simulink model "Single_phase_unipolar_mf39"  (R2023b)
settings: Solver=ode45  StartTime=0.0  StopTime=0.1  RelTol=1e-3
libraries: spsDiodeLib x4, spsIdealSwitchLib x4, spsCurrentMeasurementLib x1, spsDCVoltageSourceLib x1, spsSeriesRLCBranchLib x1, spsTriangleGeneratorLib x1, spsVoltageMeasurementLib x1, spspowerguiLib x1
settings Model: Creator=LX  LastModifiedBy=Ngsanchong
settings DataIOCC: ReturnWorkspaceOutputs=off

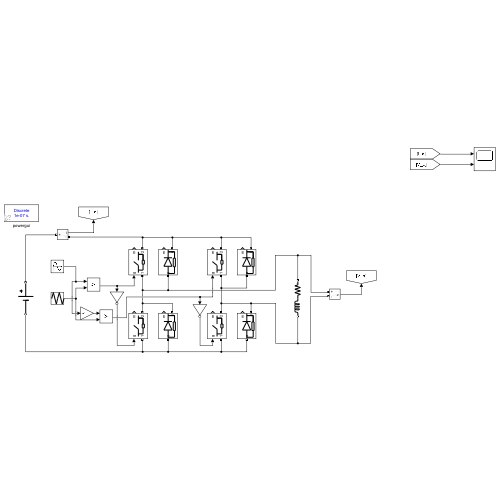
[thumbnail: Simulink's stored preview of the top-level diagram]
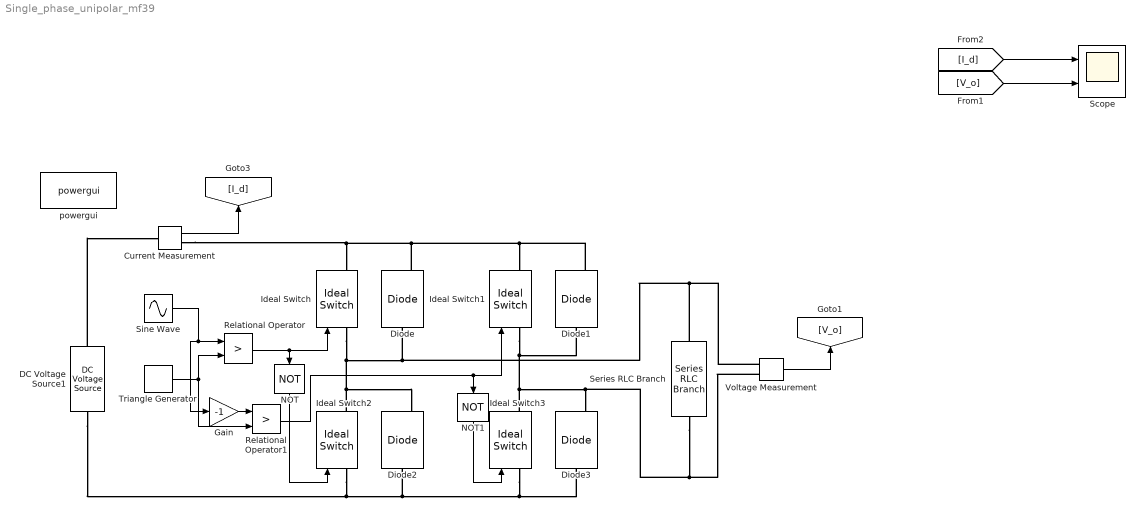
== system Single_phase_unipolar_mf39 ==
  Current Measurement : spsCurrentMeasurementLib/Current Measurement  PhasorSimulation=off  OutputType=Complex  PSBequivalent=0
  DC Voltage Source1 : spsDCVoltageSourceLib/DC Voltage Source  Amplitude=540  Measurements=None
  Diode{,1..3} (4 alike) : spsDiodeLib/Diode  Ron=0.001  Lon=0  Vf=0.8  IC=0  UseSnubber=0  Rs=500  Cs=250e-9  Measurements=on
  Gain : Gain  Gain=-1
  Ideal Switch{,1..3} (4 alike) : spsIdealSwitchLib/Ideal Switch  Ron=1e-9  Lon=0  IC=0  Rs=1e5  Cs=inf  Measurements=on
  NOT : Logic  Operator=NOT  IconShape=distinctive  AllPortsSameDT=off  OutDataTypeStr=boolean
  NOT1 : Logic  Operator=NOT  IconShape=distinctive  AllPortsSameDT=off  OutDataTypeStr=boolean
  Relational Operator : RelationalOperator  Operator=>  OutDataTypeStr=boolean  RndMeth=Simplest  InputSameDT=off
  Relational Operator1 : RelationalOperator  Operator=>  OutDataTypeStr=boolean  RndMeth=Simplest  InputSameDT=off
  Scope : Scope  NumInputPorts=2
  Series RLC Branch : spsSeriesRLCBranchLib/Series RLC Branch  LConnTagsString=__new0  RConnTagsString=__new0  BranchType=RL  Resistance=5  Inductance=5e-3  SetiL0=off  InitialCurrent=0  Capacitance=1e-6  Setx0=off  InitialVoltage=0  Measurements=None
  Sine Wave : Sin  Amplitude=0.8  Frequency=2*pi*50  SampleTime=0
  Triangle Generator : spsTriangleGeneratorLib/Triangle Generator  Freq=1950  Phase=90  Ts=0
  Voltage Measurement : spsVoltageMeasurementLib/Voltage Measurement  PhasorSimulation=off  OutputType=Complex  PSBequivalent=0
  powergui : spspowerguiLib/powergui  Priority=1  SimulationMode=Discrete  SampleTime=1e-7  frequency=60  Iterations=50  frequencyindice=0  Pbase=100e6  ErrMax=1e-4  UnitsV=kV  UnitsW=MW  buscounter=0  FunctionMessages=off  echomessages=off  EnableUseOfTLC=off  CurrentSourceSwitches=off  DisableSnubberDevices=off  DisableRonSwitches=off  DisableVfSwitches=off  DisplayEquations=off  AutomaticDiscreteSolvers=off  SolverType=Tustin/Backward Euler (TBE)  Interpol=off  ExternalGateDelay=off  methode=off  Ts=100  x0status=blocks  SPID=on  SwTol=0  HookPort=off  NonlinearTolerance=1e-4  nMaxIteration=100  ContinueOnMaxIteration=off  RestoreLinks=warning  ResistiveCurrentMeasurement=off  Frange=[0:2:500]  Ylog=off  Xlog=on  ShowGrid=off  save=off  variable=ZData  structure=0  ZoomFFT=off  StartTime=0.0  cycles=1  DisplayStyle=1  fundamental=60  FreqAxis=off  MaxFrequency=1000  frequencyindicesteady=1  RmsSteady=1  display=off
  wires:
  Sine Wave/1 -> Relational Operator/1, Gain/1
  Triangle Generator/1 -> Relational Operator1/2, Relational Operator/2
  Relational Operator/1 -> NOT/1, Ideal Switch/1
  Voltage Measurement/1 -> [V_o]
  NOT/1 -> Ideal Switch2/1
  Gain/1 -> Relational Operator1/1
  Relational Operator1/1 -> NOT1/1, Ideal Switch1/1
  NOT1/1 -> Ideal Switch3/1
  [I_d] -> Scope/1
  [V_o] -> Scope/2
  Current Measurement/1 -> [I_d]
  connections:
  Diode1/RConn1 -- Current Measurement/RConn1 -- Ideal Switch/RConn1 -- Diode/RConn1 -- Ideal Switch1/RConn1
  Ideal Switch2/RConn1 -- Diode2/RConn1 -- Ideal Switch/LConn1 -- Series RLC Branch/LConn1 -- Voltage Measurement/LConn1 -- Diode/LConn1
  Ideal Switch3/RConn1 -- Ideal Switch1/LConn1 -- Diode1/LConn1 -- Series RLC Branch/RConn1 -- Voltage Measurement/LConn2 -- Diode3/RConn1
  Ideal Switch2/LConn1 -- Diode3/LConn1 -- Ideal Switch3/LConn1 -- Diode2/LConn1 -- DC Voltage Source1/LConn1
  DC Voltage Source1/RConn1 -- Current Measurement/LConn1
